simulink model "ProbeModel_Combo"  (R2025a)
settings: Solver=ode23tb  StartTime=0.0  StopTime=1000  MaxStep=0.1  RelTol=1e-3
model workspace (MAT data in the model file):
  blend_hi = 92
  blend_lo = 90
  lower_base_wl = 80.3
  lower_top_wl = 92
  upper_base_wl = 90
  upper_top_wl = 99.6
libraries: simulink x1
settings Model: DataDictionary=FuelGaugingData.sldd  Creator=mkelley  LastModifiedBy=mkelley

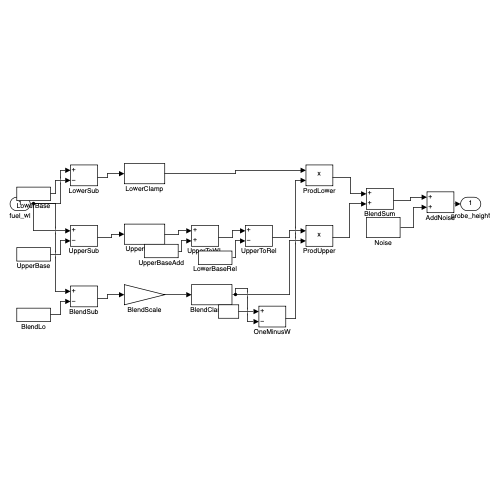
[thumbnail: Simulink's stored preview of the top-level diagram]
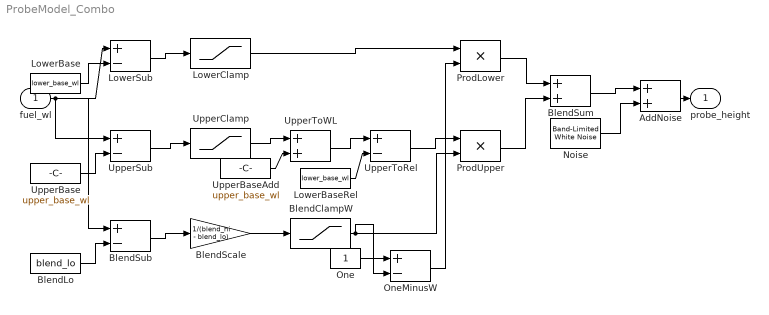
== system ProbeModel_Combo ==
  fuel_wl : Inport
  AddNoise : Sum
  BlendClampW : Saturate  UpperLimit=1  LowerLimit=0
  BlendLo : Constant  Value=blend_lo
  BlendScale : Gain  Gain=1/(blend_hi - blend_lo)
  BlendSub : Sum  Inputs=+-
  BlendSum : Sum
  LowerBase : Constant  Value=lower_base_wl
  LowerBaseRel : Constant  Value=lower_base_wl
  LowerClamp : Saturate  UpperLimit=lower_top_wl - lower_base_wl  LowerLimit=0
  LowerSub : Sum  Inputs=+-
  Noise : simulink/Sources/Band-Limited White Noise  Cov=0.0004  Ts=0.1  seed=[44721]
  One : Constant
  OneMinusW : Sum  Inputs=+-
  ProdLower : Product
  ProdUpper : Product
  UpperBase : Constant  Value=upper_base_wl
  UpperBaseAdd : Constant  Value=upper_base_wl
  UpperClamp : Saturate  UpperLimit=upper_top_wl - upper_base_wl  LowerLimit=0
  UpperSub : Sum  Inputs=+-
  UpperToRel : Sum  Inputs=+-
  UpperToWL : Sum
  probe_height : Outport
  wires:
  fuel_wl/1 -> LowerSub/1, UpperSub/1, BlendSub/1
  LowerBase/1 -> LowerSub/2
  LowerSub/1 -> LowerClamp/1
  UpperBase/1 -> UpperSub/2
  UpperSub/1 -> UpperClamp/1
  UpperClamp/1 -> UpperToWL/1
  UpperBaseAdd/1 -> UpperToWL/2
  UpperToWL/1 -> UpperToRel/1
  LowerBaseRel/1 -> UpperToRel/2
  BlendLo/1 -> BlendSub/2
  BlendSub/1 -> BlendScale/1
  BlendScale/1 -> BlendClampW/1
  UpperToRel/1 -> ProdUpper/1
  BlendClampW/1 -> ProdUpper/2, OneMinusW/2
  One/1 -> OneMinusW/1
  LowerClamp/1 -> ProdLower/1
  OneMinusW/1 -> ProdLower/2
  ProdLower/1 -> BlendSum/1
  ProdUpper/1 -> BlendSum/2
  BlendSum/1 -> AddNoise/1
  Noise/1 -> AddNoise/2
  AddNoise/1 -> probe_height/1
